simulink model "Nano_house2W"  (R2020a)
settings: Solver=ode15s  StartTime=0  StopTime=1440*7  MaxStep=1  RelTol=1e-3
libraries: Microgrid_Library x4, powerlib x1
settings Model: Creator=burmesdani  LastModifiedBy=Daniel
settings SolverCC: ZeroCrossAlgorithm=Adaptive
settings DataIOCC: ReturnWorkspaceOutputs=off
settings DebuggingCC: MaxConsecutiveZCsMsg=none  ArithmeticOperatorsInVariantConditions=warning
settings SFSimCC: SimUseLocalCustomCode=off  CustomCodeUndefinedFunction=UseInterfaceOnly
settings RTWCC: RTWUseLocalCustomCode=off
settings CodeAppCC: StateflowObjectComments=on
settings SimscapeCC: SimscapeNormalizeSystem=off

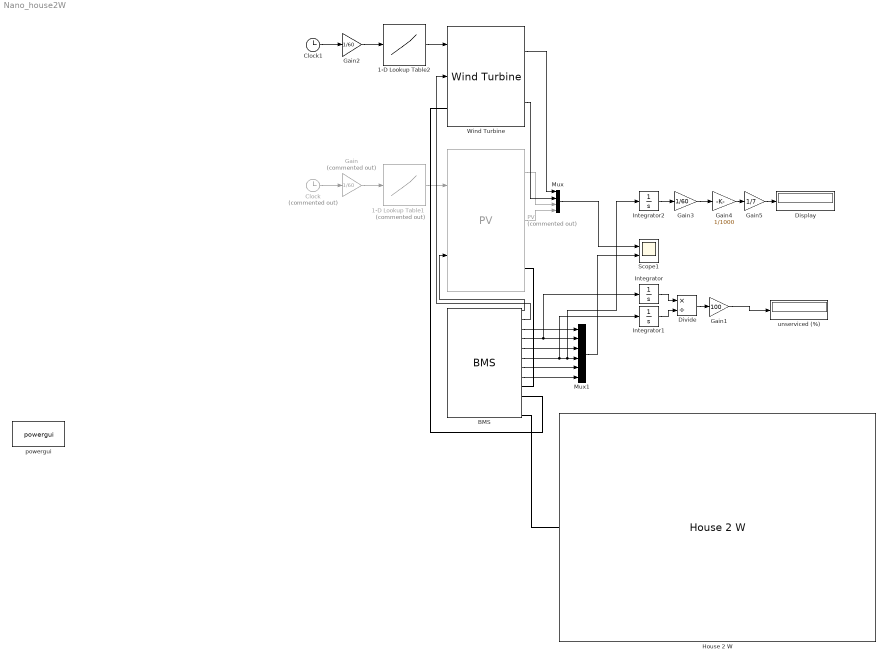
== system Nano_house2W ==
  1-D Lookup Table1 : Lookup_n-D  Commented=on  NumberOfTableDimensions=1  BreakpointsForDimension1=[ 0 1 2 3 4 5 6 7 8 9 10 11 12 13 14 15 16 17 18 19 20 21 22 23 24 25 26 27 28 29 30 31 32 33 34 35 36 37 38 39 40 41 42 43 44 45 46 47 48 49 50 51 52 53 54 55 56 57 58 59 60 61 62 63 64 65 66 67 68 69 70 71 72 73 74 75 76 77 78 79 80 81 82 83 84 85 86 87 88 89 90 91 92 93 94 95 96 97 98 99 100 101 102 103 104 105 106 107 108 109 110 111 112 113 114 115 116 117 118 119 120 121 122 123 124 125 126 127 128 129 130 131 132 133 134 135 136 137 138 139 140 141 142 143 144 145 146 147 148 149 150 151 152 153 154 155 156 157 158 159 160 161 162 163 164 165 166 167 ]  Table=|  InternalRulePriority=Speed  RndMeth=Simplest  InputSameDT=on
      | [ 0 0 0 0 0 0 0 0 24 102 216 265 347 180 457 139 14 0 0 0 0 0 0 0 0 0 0 0 0 0 0 3 102 438 606 521 454 674 419 211 67 0 0 0 0 0 0 0 0 0 0 0 0 0 0 0 20 56 105 60 86 80 111 69 23 0 0 0 0 0 0 0 0 0 0 0 0 0 0 0 20 59 207 329 494 326 573 325 86 0 0 0 0 0 0 0 0 0 0 0 0 0 0 3 79 461 545 698 753 631 556 256 120 0 0 0 0 0 0 0 0 0 0 0 0 0 0 0 23 289 555 185 105 97 116 180 25 0 0 0 0 0 0 0 0 0 0 0 0 0 0 0 26 66 128 161 217 251 160 48 40 0 0 0 0 0 0 0 
      | ]
  1-D Lookup Table2 : Lookup_n-D  NumberOfTableDimensions=1  BreakpointsForDimension1=[ 0 1 2 3 4 5 6 7 8 9 10 11 12 13 14 15 16 17 18 19 20 21 22 23 24 25 26 27 28 29 30 31 32 33 34 35 36 37 38 39 40 41 42 43 44 45 46 47 48 49 50 51 52 53 54 55 56 57 58 59 60 61 62 63 64 65 66 67 68 69 70 71 72 73 74 75 76 77 78 79 80 81 82 83 84 85 86 87 88 89 90 91 92 93 94 95 96 97 98 99 100 101 102 103 104 105 106 107 108 109 110 111 112 113 114 115 116 117 118 119 120 121 122 123 124 125 126 127 128 129 130 131 132 133 134 135 136 137 138 139 140 141 142 143 144 145 146 147 148 149 150 151 152 153 154 155 156 157 158 159 160 161 162 163 164 165 166 167 ]  Table=|  InternalRulePriority=Speed  RndMeth=Simplest  InputSameDT=on
      | [7.2
      | 6.6
      | 7.7
      | 4.6
      | 6.1
      | 5.6
      | 6.1
      | 6.6
      | 5.6
      | 5.6
      | 5.6
      | 5.1
      | 9.2
      | 7.7
      | 6.6
      | 6.1
      | 6.6
      | 6.1
      | 5.6
      | 6.1
      | 4.1
      | 2.5
      | 1.5
      | 3
      | 3.6
      | 4.1
      | 3
      | 3
      | 2
      | 1
      | 1.5
      | 1.5
      | 3
      | 4.6
      | 4.6
      | 5.1
      | 5.1
      | 7.7
      | 8.7
      | 6.6
      | 7.2
      | 6.1
      | 6.6
      | 6.1
      | 5.6
      | 6.1
      | 7.7
      | 8.7
      | 9.2
      | 8.7
      | 8.2
      | 7.7
      | 8.7
      | 9.2
      | 10.8
      | 9.2
      | 8.7
      | 9.2
      | 9.2
      | 12.3
      | 9.7
      | 8.2
      | 5.1
      | 7.2
      | 8.2
      | 7.2
      | 8.2
      | 6.6
      | 7.2
      | 5.6
      | 5.6
      | 5.6
      | 4.1
      | 5.1
      | 5.6
      | 5.1
      | 3
      | 4.1
      | 2.5
      | 1.5
      | 0.5
      | 1
      | 0
      | 6.6
      | 9.2
      | 11.3
      | 11.8
      | 8.2
      | 7.2
      | 6.1
      | 6.1
      | 4.6
      | 4.6
      | 4.1
      | 4.1
      | 3.6
      | 3
      | 2
      | 2
      | 2
      | 2
      | 2.5
      | 2
      | 2
      | 1.5
      | 1
      | 0
      | 2.5
      | 2.5
      | 3
      | 3.6
      | 3.6
      | 4.1
      | 4.6
      | 3.6
      | 2.5
      | 2.5
      | 2.5
      | 1.5
      | 5.1
      | 4.6
      | 5.1
      | 7.2
      | 6.6
      | 8.2
      | 5.6
      | 4.6
      | 2.5
      | 1
      | 1
      | 5.1
      | 10.3
      | 11.3
      | 11.3
      | 11.8
      | 10.8
      | 9.7
      | 9.2
      | 9.2
      | 8.2
      | 8.2
      | 7.7
      | 6.6
      | 7.2
      | 3.6
      | 5.6
      | 2
      | 3
      | 2.5
      | 2
      | 2.5
      | 2
      | 2
      | 2
      | 2
      | 2.5
      | 3
      | 3
      | 5.6
      | 7.7
      | 9.2
      | 10.3
      | 11.8
      | 15.4
      | 15.4
      | 15.4
      | 14.9
      | 12.8]
  BMS : Microgrid_Library/BMS  v=240  c=80
  Clock : Clock  Commented=on
  Clock1 : Clock
  Display : Display
  Divide : Product  Inputs=*/
  Gain : Gain  Commented=on  Gain=1/60
  Gain1 : Gain  Gain=100
  Gain2 : Gain  Gain=1/60
  Gain3 : Gain  Gain=1/60
  Gain4 : Gain  Gain=1/1000
  Gain5 : Gain  Gain=1/7
  House 2 W : Microgrid_Library/House 2 W  V=240  t=60  K_L1_W=40  K_L1_On_1=63000  K_L1_Off_1=72600  K_L1_On_2=0  K_L1_Off_2=0  Dishwasher_W=1200  Dishwasher_On=72000  Fridge_W=150  T_Initial=1.9  T_Low=1  T_High=2.4  Jug_W=1500  Jug_On_1=25200  Jug_On_2=64200  Jug_On_3=0  Toaster_W=900  Toaster_On_1=23400  Toaster_On_2=27120  N_Elements=4  Oven_On_1=63600  Oven_Off_1=67200  Shower_On_a=21720  Shower_L_a=240  Shower_On_b=23640  Shower_L_b=300  Shower_On_c=0  Shower_L_c=0  K_L3_W=60  K_L3_On_1=21480  K_L3_Off_1=22140  K_L3_On_2=23580  K_L3_Off_2=24780  HW_W=2000  M=177  D=0.488  L=1.72  Ti=7  Ta=20  T_Low_WH=58  T_High_WH=61  Clock_1_W=5  Lamp_1_W=18  L1_On_1=79740  L1_Off_1=83040  L1_On_2=0  L1_Off_2=0  K_L4_W=24  K_L4_On_1=21000  K_L4_Off_1=27360  Clock_2_W=6  Lamp_2_W=24  L2_On_1=26820  L2_Off_1=29160  L2_On_2=73800  L2_Off_2=76800  K_L5_W=40  K_L5_On_1=28800  K_L5_Off_1=30240  K_L5_On_2=72300  K_L5_Off_2=83880  Phone_C_1_W=3  Phone_C_1_On_a=0  Phone_C_1_Off_a=35700  Phone_C_1_On_b=76800  Phone_C_1_Off_b=86400  Phone_C_2_W=7  Phone_C_2_On_a=0  Phone_C_2_Off_a=35760  Phone_C_2_On_b=76800  Phone_C_2_Off_b=86400  Phone_C_3_W=5  Phone_C_3_On_a=0  Phone_C_3_Off_a=35700  Phone_C_3_On_b=77040  Phone_C_3_Off_b=86400  Laptop_C_1_W=55  Laptop_C_1_On_a=76800  Laptop_C_1_Off_a=86400  Laptop_C_2_W=65  Laptop_C_2_On_a=0  Laptop_C_2_Off_a=28500  Laptop_C_2_On_b=77160  Laptop_C_2_Off_b=86400  Lamp_3_W=60  L3_On_1=21600  L3_Off_1=27000  L3_On_2=62760  L3_Off_2=83220  K_L6_W=60  K_L6_On_1=68400  K_L6_Off_1=70200  Heater_W=1800  Heater_On_1=62040  Heater_Off_1=68640  Stereo_W=100  Stereo_On_1=42480  Stereo_Off_1=58200  TV_W=500  TV_On_1=21900  TV_Off_1=26580  TV_On_2=63000  TV_Off_2=73200
  Integrator : Integrator
  Integrator1 : Integrator
  Integrator2 : Integrator
  Mux : Mux
  Mux1 : Mux  Inputs=6
  PV : Microgrid_Library/PV  Commented=on  P=10
  Scope1 : Scope  NumInputPorts=2
  Wind Turbine : Microgrid_Library/Wind Turbine  V=240  W=2000
  powergui : powerlib/powergui  Priority=1  SimulationMode=Continuous  SampleTime=50e-6  frequency=60  Iterations=50  frequencyindice=0  Pbase=100e6  ErrMax=1e-4  UnitsV=kV  UnitsW=MW  buscounter=0  FunctionMessages=off  echomessages=off  EnableUseOfTLC=off  CurrentSourceSwitches=off  DisableSnubberDevices=off  DisableRonSwitches=off  DisableVfSwitches=off  DisplayEquations=off  AutomaticDiscreteSolvers=off  SolverType=Tustin/Backward Euler (TBE)  Interpol=off  ExternalGateDelay=off  methode=off  Ts=100  x0status=blocks  SPID=on  SwTol=0  HookPort=off  NonlinearTolerance=1e-4  nMaxIteration=100  ContinueOnMaxIteration=off  RestoreLinks=warning  ResistiveCurrentMeasurement=off  Frange=[0:2:500]  Ylog=off  Xlog=on  ShowGrid=off  save=off  variable=ZData  structure=0  ZoomFFT=off  StartTime=0.0  cycles=1  DisplayStyle=1  fundamental=60  FreqAxis=off  MaxFrequency=1000  frequencyindicesteady=1  RmsSteady=1  display=off
  unserviced (%) : Display
  wires:
  1-D Lookup Table1/1 -> PV/1
  Gain/1 -> 1-D Lookup Table1/1
  Clock/1 -> Gain/1
  PV/1 -> Mux/3
  PV/2 -> Mux/4
  BMS/1 -> PV/2
  BMS/3 -> Mux1/1
  BMS/4 -> Integrator/1, Mux1/2
  BMS/5 -> Mux1/3
  BMS/7 -> Mux1/5
  BMS/8 -> Mux1/6
  Mux/1 -> Scope1/1
  BMS/6 -> Integrator1/1, Integrator2/1, Mux1/4
  Mux1/1 -> Scope1/2
  Integrator/1 -> Divide/1
  Integrator1/1 -> Divide/2
  Divide/1 -> Gain1/1
  Gain1/1 -> unserviced (%)/1
  Gain2/1 -> 1-D Lookup Table2/1
  Clock1/1 -> Gain2/1
  1-D Lookup Table2/1 -> Wind Turbine/1
  BMS/2 -> Wind Turbine/2
  Wind Turbine/2 -> Mux/2
  Wind Turbine/1 -> Mux/1
  Integrator2/1 -> Gain3/1
  Gain3/1 -> Gain4/1
  Gain4/1 -> Gain5/1
  Gain5/1 -> Display/1
  connections:
  BMS/RConn1 -- PV/RConn1
  BMS/RConn4 -- House 2 W/LConn1
  BMS/RConn2 -- Wind Turbine/LConn1
